simulink model "TV_sim_with_sine"  (R2015a)
settings: Solver=ode45  StartTime=0.0  StopTime=30  RelTol=1e-3
libraries: dspsrcs4 x3, dspsnks4 x1
settings Model: Creator=ekulasek  LastModifiedBy=ekulasek

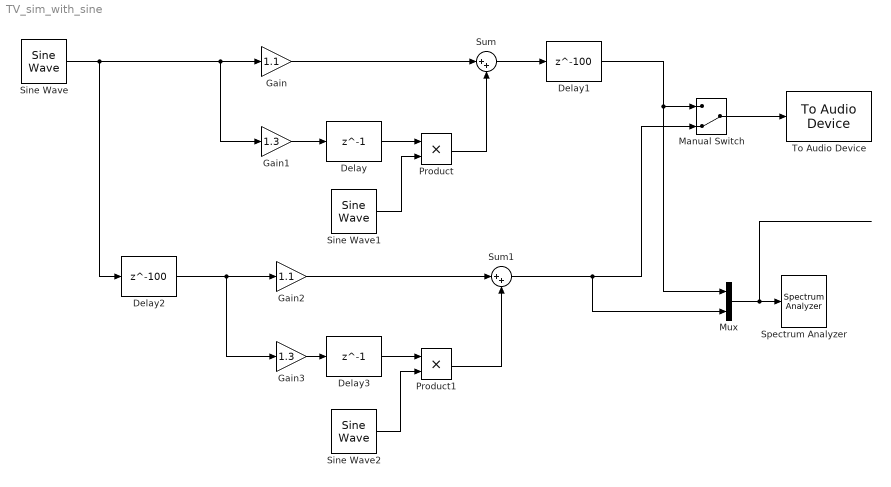
== system TV_sim_with_sine ==
  Delay : Delay  DelayLength=1  InputProcessing=Columns as channels (frame based)
  Delay1 : Delay  DelayLength=100  InputProcessing=Columns as channels (frame based)
  Delay2 : Delay  DelayLength=100  InputProcessing=Columns as channels (frame based)
  Delay3 : Delay  DelayLength=1  InputProcessing=Columns as channels (frame based)
  Gain : Gain  Gain=1.1
  Gain1 : Gain  Gain=1.3
  Gain2 : Gain  Gain=1.1
  Gain3 : Gain  Gain=1.3
  Manual Switch : ManualSwitch  CurrentSetting=0
  Mux : Mux  Inputs=2
  Product : Product  OutDataTypeStr=Inherit: Same as first input
  Product1 : Product  OutDataTypeStr=Inherit: Same as first input
  Sine Wave : dspsrcs4/Sine Wave  Amplitude=1  Frequency=100  Phase=0  SampleMode=Discrete  OutComplex=Real  CompMethod=Trigonometric fcn  TableSize=Speed  SampleTime=1/1000  SamplesPerFrame=1  ResetState=Restart at time zero  dataType=double  wordLen=16  udDataType=sfix(16)  fracBitsMode=Best precision  numFracBits=15  OutDataTypeStr=double  LastOutDataTypeStr=double
  Sine Wave1 : dspsrcs4/Sine Wave  Amplitude=2  Frequency=385  Phase=0  SampleMode=Discrete  OutComplex=Real  CompMethod=Trigonometric fcn  TableSize=Speed  SampleTime=1/1000  SamplesPerFrame=1  ResetState=Restart at time zero  dataType=double  wordLen=16  udDataType=sfix(16)  fracBitsMode=Best precision  numFracBits=15  OutDataTypeStr=double  LastOutDataTypeStr=double
  Sine Wave2 : dspsrcs4/Sine Wave  Amplitude=2  Frequency=385  Phase=0  SampleMode=Discrete  OutComplex=Real  CompMethod=Trigonometric fcn  TableSize=Speed  SampleTime=1/1000  SamplesPerFrame=1  ResetState=Restart at time zero  dataType=double  wordLen=16  udDataType=sfix(16)  fracBitsMode=Best precision  numFracBits=15  OutDataTypeStr=double  LastOutDataTypeStr=double
  Spectrum Analyzer : SpectrumAnalyzer
  Sum : Sum  Inputs=|++
  Sum1 : Sum  Inputs=|++
  To Audio Device : dspsnks4/To Audio Device  deviceName=Default  inheritSampleRate=on  sampleRate=44100  deviceDatatype=Determine from input data type  autoBufferSize=on  bufferSize=4096  queueDuration=1.0  defaultOutputChannelMapping=on  outputChannelMapping=1:32  outputNumUnderrunSamples=off
  wires:
  Gain/1 -> Sum/1
  Gain1/1 -> Delay/1
  Sum/1 -> Delay1/1
  Sine Wave/1 -> Gain1/1, Gain/1, Delay2/1
  Gain2/1 -> Sum1/1
  Gain3/1 -> Delay3/1
  Delay2/1 -> Gain3/1, Gain2/1
  Manual Switch/1 -> To Audio Device/1
  Delay1/1 -> Mux/1, Manual Switch/1
  Sum1/1 -> Mux/2, Manual Switch/2
  Delay/1 -> Product/1
  Product/1 -> Sum/2
  Sine Wave1/1 -> Product/2
  Delay3/1 -> Product1/1
  Sine Wave2/1 -> Product1/2
  Product1/1 -> Sum1/2
  Mux/1 -> Spectrum Analyzer/1
